simulink model "first"  (R2020b)
settings: Solver=VariableStepAuto  StartTime=0.0  StopTime=10.0  RelTol=1e-3
libraries: cstblocks x3
settings Model: Creator=Mah  LastModifiedBy=Mah

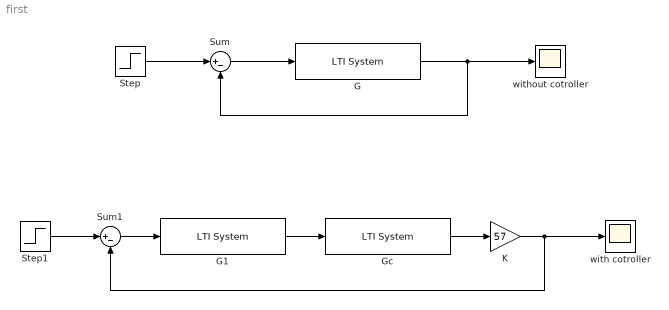
== system first ==
  G : cstblocks/LTI System  sys=tf(64.11 , [1 36.42 0])  IC=[]
  G1 : cstblocks/LTI System  sys=tf(64.11 , [1 36.42 0])  IC=[]
  Gc : cstblocks/LTI System  sys=tf([1 40] , [1 87.6383])  IC=[]
  K : Gain  Gain=57
  Step : Step  Time=0  SampleTime=0
  Step1 : Step  Time=0  SampleTime=0
  Sum : Sum  Inputs=|+-
  Sum1 : Sum  Inputs=|+-
  with cotroller : Scope
  without cotroller : Scope
  wires:
  Sum/1 -> G/1
  G/1 -> Sum/2, without cotroller/1
  Step/1 -> Sum/1
  G1/1 -> Gc/1
  Gc/1 -> K/1
  Sum1/1 -> G1/1
  Step1/1 -> Sum1/1
  K/1 -> with cotroller/1, Sum1/2
